simulink model "Modelo_Motor_Minimos_Quadrados"  (R2023b)
settings: Solver=FixedStepAuto  StartTime=0.0  StopTime=7  FixedStep=T  RelTol=1e-3
model workspace (MAT data in the model file):
  B = 0.0928996133407
  Cmn = 479.991198073
  I = 3000
  Ian = 260.13143483
  J = 0.56
  Kf = 1.91586963478
  La = 0.0014
  N = 3000
  Pele = 104052.573932
  Pmec = 95000
  Ra = 0.08
  T = 0.00175
  Te = 0.0175
  Tm = 6.02801217209
  Vn = 400
  Wn = 197.920296
libraries: simulink x4
settings Model: Creator=USER  LastModifiedBy=USER

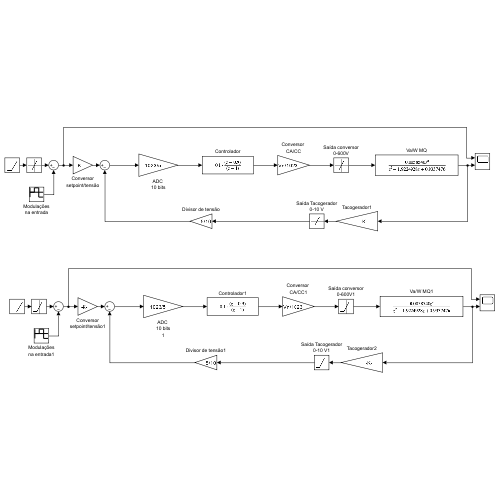
[thumbnail: Simulink's stored preview of the top-level diagram]
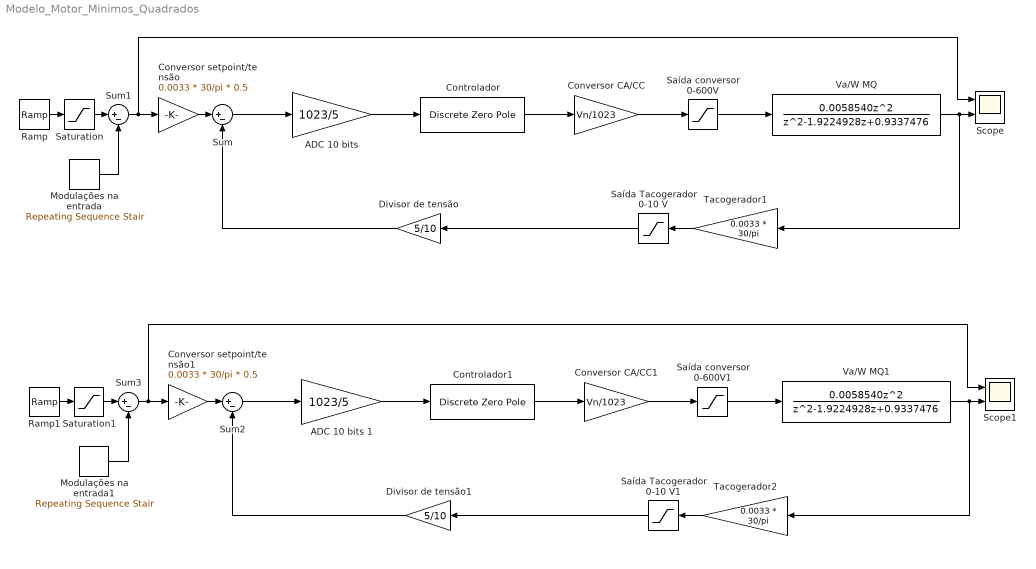
== system Modelo_Motor_Minimos_Quadrados ==
  "ADC 10 bits " : Gain  Gain=1023/5
  ADC 10 bits 1 : Gain  Gain=1023/5
  Controlador : DiscreteZeroPole  Zeros=[0.9]  Poles=[1]  Gain=0.1  SampleTime=-1
  Controlador1 : DiscreteZeroPole  Zeros=[0.9]  Poles=[1]  Gain=0.1  SampleTime=-1
  Conversor setpoint/tensão : Gain  Gain=0.0033 * 30/pi * 0.5
  Conversor setpoint/tensão1 : Gain  Gain=0.0033 * 30/pi * 0.5
  Conversor CA/CC : Gain  Gain=Vn/1023
  Conversor CA/CC1 : Gain  Gain=Vn/1023
  Divisor de tensão : Gain  Gain=5/10
  Divisor de tensão1 : Gain  Gain=5/10
  Modulações na entrada : simulink/Sources/Repeating Sequence Stair  OutValues=[0 50 -50].'  tsamp=1143 * T  OutMin=[]  OutMax=[]  OutDataTypeStr=double  OutputDataTypeScalingMode=double  OutDataType=fixdt(0,8)  ConRadixGroup=Best Precision: Vector-wise  OutScaling=2^-12
  Modulações na entrada1 : simulink/Sources/Repeating Sequence Stair  OutValues=[0 50 -50].'  tsamp=1143 * T  OutMin=[]  OutMax=[]  OutDataTypeStr=double  OutputDataTypeScalingMode=double  OutDataType=fixdt(0,8)  ConRadixGroup=Best Precision: Vector-wise  OutScaling=2^-12
  Ramp : simulink/Sources/Ramp  slope=Wn*20  start=0  InitialOutput=0
  Ramp1 : simulink/Sources/Ramp  slope=Wn*20  start=0  InitialOutput=0
  Saturation : Saturate  UpperLimit=Wn
  Saturation1 : Saturate  UpperLimit=Wn
  Saída Tacogerador 0-10 V : Saturate  UpperLimit=10  LowerLimit=0
  Saída Tacogerador 0-10 V1 : Saturate  UpperLimit=10  LowerLimit=0
  Saída conversor 0-600V : Saturate  UpperLimit=600  LowerLimit=0
  Saída conversor 0-600V1 : Saturate  UpperLimit=600  LowerLimit=0
  Scope : Scope  NumInputPorts=2
  Scope1 : Scope  NumInputPorts=2
  Sum{,1..3} (4 alike) : Sum  Inputs=|+-
  Tacogerador1 : Gain  Gain=0.0033 * 30/pi
  Tacogerador2 : Gain  Gain=0.0033 * 30/pi
  Va/W MQ : DiscreteTransferFcn  Numerator=[0.0058540, 0, 0]  Denominator=[1, -1.9224928, 0.9337476]
  Va/W MQ1 : DiscreteTransferFcn  Numerator=[0.0058540, 0, 0]  Denominator=[1, -1.9224928, 0.9337476]
  wires:
  Saída Tacogerador 0-10 V/1 -> Divisor de tensão/1
  Modulações na entrada/1 -> Sum1/2
  Saturation/1 -> Sum1/1
  Conversor setpoint/tensão/1 -> Sum/1
  Sum/1 -> "ADC 10 bits "/1
  Divisor de tensão/1 -> Sum/2
  Conversor CA/CC/1 -> Saída conversor 0-600V/1
  "ADC 10 bits "/1 -> Controlador/1
  Tacogerador1/1 -> Saída Tacogerador 0-10 V/1
  Saída conversor 0-600V/1 -> Va/W MQ/1
  Va/W MQ/1 -> Tacogerador1/1, Scope/2
  Sum1/1 -> Scope/1, Conversor setpoint/tensão/1
  Ramp/1 -> Saturation/1
  Controlador/1 -> Conversor CA/CC/1
  Controlador1/1 -> Conversor CA/CC1/1
  Conversor setpoint/tensão1/1 -> Sum2/1
  Saturation1/1 -> Sum3/1
  Saída Tacogerador 0-10 V1/1 -> Divisor de tensão1/1
  Va/W MQ1/1 -> Tacogerador2/1, Scope1/2
  ADC 10 bits 1/1 -> Controlador1/1
  Ramp1/1 -> Saturation1/1
  Sum2/1 -> ADC 10 bits 1/1
  Modulações na entrada1/1 -> Sum3/2
  Tacogerador2/1 -> Saída Tacogerador 0-10 V1/1
  Conversor CA/CC1/1 -> Saída conversor 0-600V1/1
  Saída conversor 0-600V1/1 -> Va/W MQ1/1
  Divisor de tensão1/1 -> Sum2/2
  Sum3/1 -> Scope1/1, Conversor setpoint/tensão1/1
